simulink model "atividadepratica2"  (R2021b)
settings: Solver=VariableStepAuto  StartTime=0.0  StopTime=100  RelTol=1e-3
libraries: simulink x1
settings Model: Creator=a2103303  LastModifiedBy=a2103303

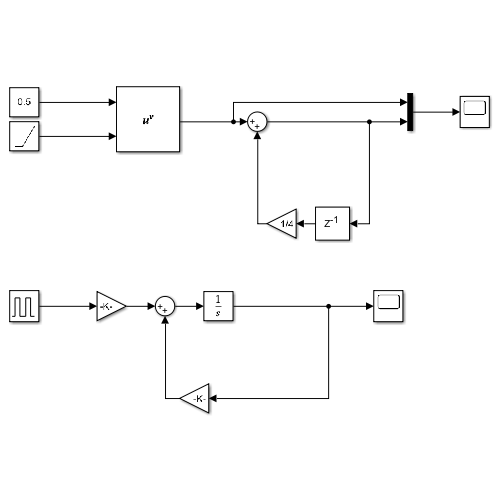
[thumbnail: Simulink's stored preview of the top-level diagram]
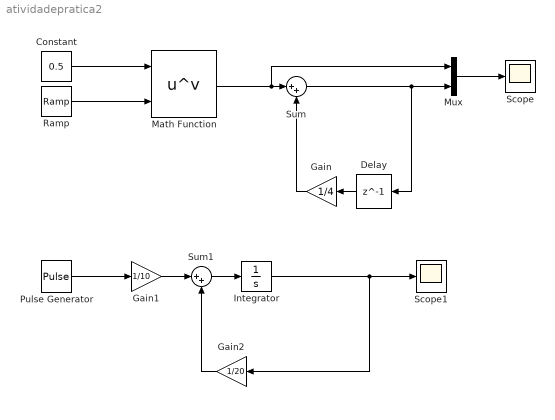
== system atividadepratica2 ==
  Constant : Constant  Value=0.5
  Delay : Delay  DelayLength=1  InitialCondition=8
  Gain : Gain  Gain=1/4
  Gain1 : Gain  Gain=1/10
  Gain2 : Gain  Gain=1/20
  Integrator : Integrator
  Math Function : Math  Operator=pow  SaturateOnIntegerOverflow=on
  Mux : Mux  Inputs=2
  Pulse Generator : DiscretePulseGenerator  PulseType=Time based  Period=10  PulseWidth=5
  Ramp : simulink/Sources/Ramp  slope=1  start=0  InitialOutput=0
  Scope : Scope
  Scope1 : Scope
  Sum : Sum  Inputs=|++
  Sum1 : Sum  Inputs=|++
  wires:
  Ramp/1 -> Math Function/2
  Constant/1 -> Math Function/1
  Math Function/1 -> Sum/1, Mux/1
  Mux/1 -> Scope/1
  Sum/1 -> Delay/1, Mux/2
  Delay/1 -> Gain/1
  Gain/1 -> Sum/2
  Sum1/1 -> Integrator/1
  Integrator/1 -> Scope1/1, Gain2/1
  Gain2/1 -> Sum1/2
  Pulse Generator/1 -> Gain1/1
  Gain1/1 -> Sum1/1
